simulink model "TransmissionLine"  (R2025a)
settings: Solver=ode15s  StartTime=0.0  StopTime=0.2  RelTol=1e-3
libraries: spsFourierLib x6, dspfdesign x6, spsDistributedParametersLineLib x2, spsThreePhaseVIMeasurementLib x2, spsThreePhaseBreakerLib x2, spsThreePhaseSourceLib x2, simulink_extras x1, spsOnDelayLib x1, spsThreePhaseFaultLib x1, sps_lib x1
settings Model: Creator=monji  LastModifiedBy=monji

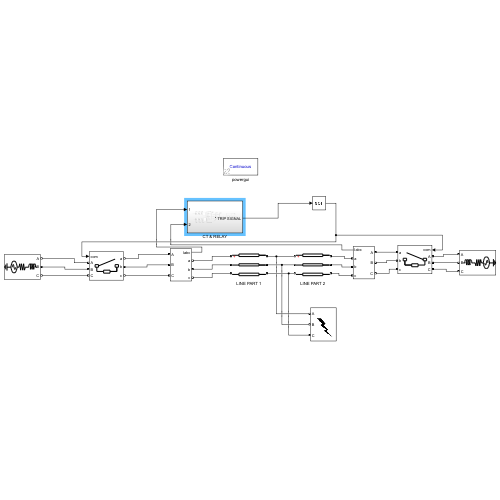
[thumbnail: Simulink's stored preview of the top-level diagram]
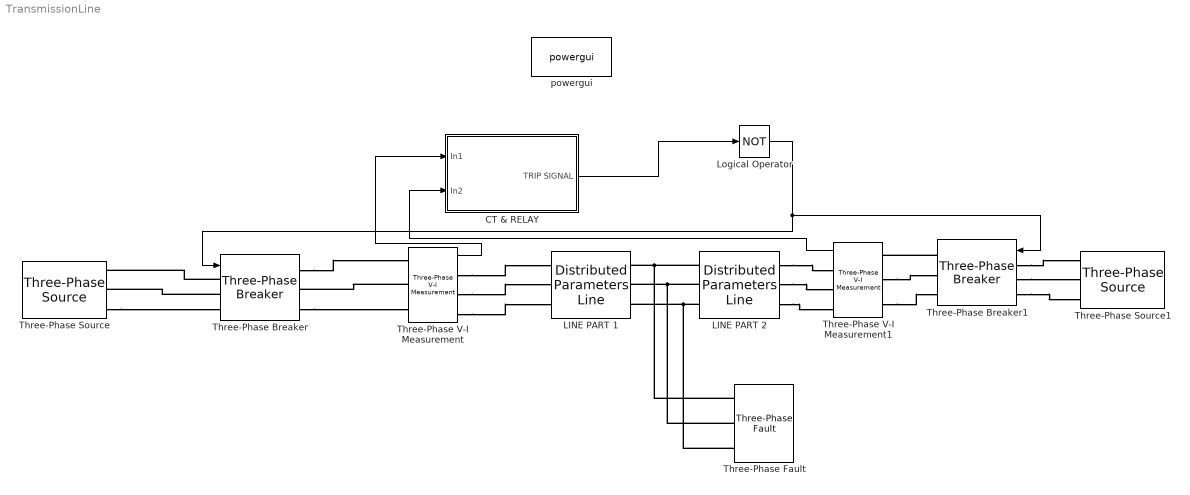
== system TransmissionLine ==
  CT & RELAY : Subsystem
  LINE PART 1 : spsDistributedParametersLineLib/Distributed Parameters Line  Phases=3  Length=10  Frequency=50  Resistance=[0.045531917 0.151489359 ]  Inductance=[0.0006176566224 0.001533982723]  Capacitance=[0.013e-8 0.0085e-8]  x1=[1.46385157011448e-06 84909.030148672 84909.030146414;314.159265358979 314.159265358979 314.159265358979;-0.0832984052830537 0.256881061681218 -1.31391526508876]  x2=[1.4638153564349e-06 84909.0444627924 84909.0444605344;314.159265358979 314.159265358979 314.159265358979;-0.0832705183654309 0.256879998490702 -1.31391632827928]  x3=[3.47740712938383e-10 38.9054582092484 38.90545820819;314.159265358979 314.159265358979 314.159265358979;-0.0653475125454102 0.255989829496242 -1.31480649727325]  x4=[3.43279937985723e-10 38.9903495109087 38.9903495098979;314.159265358979 314.159265358979 314.159265358979;-0.109935333243445 0.256879998680736 -1.31391632808959]  x5=3.61093521757176e-06  V1=[1.464e-06 8.491e+04 8.491e+04;314.2 314.2 314.2;-0.0833 0.2569 -1.314]  V2=[1.464e-06 8.491e+04 8.491e+04;314.2 314.2 314.2;-0.08327 0.2569 -1.314]  I1=[3.477e-10 38.91 38.91;314.2 314.2 314.2;-0.06535 0.256 -1.315]  I2=[3.433e-10 38.99 38.99;314.2 314.2 314.2;-0.1099 0.2569 -1.314]  nHarmo=1  Measurements=None  Decoupling=off  VsMag0=0  VrMag0=0  VsAngle0=0  VrAngle0=0  IsMag0=0  IrMag0=0  IsAngle0=0  IrAngle0=0
      settings: LibrarySourceBlock=sps_lib/Power Grid Elements/Distributed Parameters Line
  LINE PART 2 : spsDistributedParametersLineLib/Distributed Parameters Line  Phases=3  Length=10  Frequency=50  Resistance=[0.045531917 0.151489359 ]  Inductance=[0.0006176566224 0.001533982723]  Capacitance=[0.013e-8 0.0085e-8]  x1=[1.4638153564349e-06 84909.0444627924 84909.0444605344;314.159265358979 314.159265358979 314.159265358979;-0.0832705183654309 0.256879998490702 -1.31391632827928]  x2=[1.46379725002201e-06 84909.0301487049 84909.0301464468;314.159265358979 314.159265358979 314.159265358979;-0.0832565743891926 0.256881061681343 -1.31391526508863]  x3=[3.46588857006348e-10 38.99034951986 38.9903495188265;314.159265358979 314.159265358979 314.159265358979;-0.0822700055886377 0.256879998301002 -1.31391632846952]  x4=[3.4292641339421e-10 38.9054582002993 38.9054581992604;314.159265358979 314.159265358979 314.159265358979;-0.100050154115277 0.255989829876863 -1.31480649689257]  x5=3.61093521757176e-06  V1=[1.464e-06 8.491e+04 8.491e+04;314.2 314.2 314.2;-0.08327 0.2569 -1.314]  V2=[1.464e-06 8.491e+04 8.491e+04;314.2 314.2 314.2;-0.08326 0.2569 -1.314]  I1=[3.466e-10 38.99 38.99;314.2 314.2 314.2;-0.08227 0.2569 -1.314]  I2=[3.429e-10 38.91 38.91;314.2 314.2 314.2;-0.1001 0.256 -1.315]  nHarmo=1  Measurements=None  Decoupling=off  VsMag0=0  VrMag0=0  VsAngle0=0  VrAngle0=0  IsMag0=0  IrMag0=0  IsAngle0=0  IrAngle0=0
      settings: LibrarySourceBlock=sps_lib/Power Grid Elements/Distributed Parameters Line
  Logical Operator : Logic  Operator=NOT  AllPortsSameDT=off  OutDataTypeStr=boolean
  Three-Phase V-I Measurement : spsThreePhaseVIMeasurementLib/Three-Phase V-I Measurement  VoltageMeasurement=no  SetLabelV=off  LabelV=Vabc  Vpu=off  VpuLL=off  CurrentMeasurement=yes  SetLabelI=off  LabelI=Iabc  Ipu=off  Pbase=100e6  Vbase=500e3  OutputType=Complex  PhasorSimulation=off  PSBequivalent=0
  Three-Phase V-I Measurement1 : spsThreePhaseVIMeasurementLib/Three-Phase V-I Measurement  VoltageMeasurement=no  SetLabelV=off  LabelV=Vabc  Vpu=off  VpuLL=off  CurrentMeasurement=yes  SetLabelI=off  LabelI=Iabc  Ipu=off  Pbase=100e6  Vbase=500e3  OutputType=Complex  PhasorSimulation=off  PSBequivalent=0
  Three-Phase Breaker : spsThreePhaseBreakerLib/Three-Phase Breaker  InitialState=open  SwitchA=on  SwitchB=on  SwitchC=on  SwitchTimes="[1/60  5/60]"  External=on  BreakerResistance=0.001  SnubberResistance=1e6  SnubberCapacitance=inf  Measurements=None
  Three-Phase Breaker1 : spsThreePhaseBreakerLib/Three-Phase Breaker  InitialState=open  SwitchA=on  SwitchB=on  SwitchC=on  SwitchTimes="[1/60  5/60]"  External=on  BreakerResistance=0.001  SnubberResistance=1e6  SnubberCapacitance=inf  Measurements=None
  Three-Phase Fault : spsThreePhaseFaultLib/Three-Phase Fault  InitialStates=0  FaultA=off  FaultB=on  FaultC=on  GroundFault=off  SwitchTimes=[0.05 0.1]  External=off  SwitchStatus=NaN  FaultResistance=5  GroundResistance=0.01  SnubberResistance=1e6  SnubberCapacitance=inf  Measurements=None
  Three-Phase Source : spsThreePhaseSourceLib/Three-Phase Source  InternalConnection=Yg  VoltagePhases=off  Voltage=132e3  PhaseAngle=0  Voltage_phases=[25e3 25e3 25e3]/sqrt(3)  PhaseAngles_phases=[0 -120 +120]  Frequency=50  NonIdealSource=on  SpecifyImpedance=on  Resistance=0.8929  Inductance=16.58e-3  ShortCircuitLevel=2e9  BaseVoltage=25e3  XRratio=7  BusType=swing  Pref=10e3  Qref=0  Prefabc=[10e3, 10e3, 10e3]  Qrefabc=[0, 0, 0]  Qmin=-inf  Qmax=inf
  Three-Phase Source1 : spsThreePhaseSourceLib/Three-Phase Source  InternalConnection=Yg  VoltagePhases=off  Voltage=132e3  PhaseAngle=0  Voltage_phases=[25e3 25e3 25e3]/sqrt(3)  PhaseAngles_phases=[0 -120 +120]  Frequency=50  NonIdealSource=on  SpecifyImpedance=on  Resistance=0.8929  Inductance=16.58e-3  ShortCircuitLevel=1e9  BaseVoltage=25e3  XRratio=7  BusType=swing  Pref=10e3  Qref=0  Prefabc=[10e3, 10e3, 10e3]  Qrefabc=[0, 0, 0]  Qmin=-inf  Qmax=inf
  powergui : sps_lib/powergui  Priority=1  SimulationMode=Continuous  SampleTime=50e-6  frequency=60  Iterations=50  frequencyindice=50  Pbase=100e6  ErrMax=1e-4  UnitsV=kV  UnitsW=MW  buscounter=0  FunctionMessages=off  echomessages=off  EnableUseOfTLC=off  CurrentSourceSwitches=off  DisableSnubberDevices=off  DisableRonSwitches=off  DisableVfSwitches=off  DisplayEquations=off  AutomaticDiscreteSolvers=off  SolverType=Tustin/Backward Euler (TBE)  Interpol=off  ExternalGateDelay=off  methode=off  Ts=100  x0status=blocks  SPID=on  SwTol=0  HookPort=off  NonlinearTolerance=1e-4  nMaxIteration=100  ContinueOnMaxIteration=off  RestoreLinks=warning  ResistiveCurrentMeasurement=off  Frange=[0:2:500]  Ylog=off  Xlog=on  ShowGrid=off  save=off  variable=ZData  structure=0  ZoomFFT=off  StartTime=0.0  cycles=1  DisplayStyle=1  fundamental=60  FreqAxis=off  MaxFrequency=1000  frequencyindicesteady=1  RmsSteady=1  display=off
  wires:
  Three-Phase V-I Measurement/1 -> CT & RELAY/1(In1)
  Three-Phase V-I Measurement1/1 -> CT & RELAY/2(In2)
  CT & RELAY/1(TRIP SIGNAL) -> Logical Operator/1
  Logical Operator/1 -> Three-Phase Breaker1/1, Three-Phase Breaker/1
  connections:
  Three-Phase V-I Measurement/RConn1 -- LINE PART 1/LConn1
  Three-Phase V-I Measurement/RConn2 -- LINE PART 1/LConn2
  Three-Phase V-I Measurement/RConn3 -- LINE PART 1/LConn3
  LINE PART 2/LConn1 -- Three-Phase Fault/LConn1 -- LINE PART 1/RConn1
  LINE PART 2/LConn2 -- Three-Phase Fault/LConn2 -- LINE PART 1/RConn2
  LINE PART 2/LConn3 -- Three-Phase Fault/LConn3 -- LINE PART 1/RConn3
  LINE PART 2/RConn1 -- Three-Phase V-I Measurement1/RConn1
  LINE PART 2/RConn2 -- Three-Phase V-I Measurement1/RConn2
  LINE PART 2/RConn3 -- Three-Phase V-I Measurement1/RConn3
  Three-Phase Breaker/LConn1 -- Three-Phase Source/RConn1
  Three-Phase Breaker/LConn2 -- Three-Phase Source/RConn2
  Three-Phase Source/RConn3 -- Three-Phase Breaker/LConn3
  Three-Phase Breaker/RConn1 -- Three-Phase V-I Measurement/LConn1
  Three-Phase V-I Measurement/LConn2 -- Three-Phase Breaker/RConn2
  Three-Phase Breaker/RConn3 -- Three-Phase V-I Measurement/LConn3
  Three-Phase Breaker1/RConn1 -- Three-Phase V-I Measurement1/LConn1
  Three-Phase V-I Measurement1/LConn2 -- Three-Phase Breaker1/RConn2
  Three-Phase V-I Measurement1/LConn3 -- Three-Phase Breaker1/RConn3
  Three-Phase Breaker1/LConn1 -- Three-Phase Source1/RConn1
  Three-Phase Breaker1/LConn2 -- Three-Phase Source1/RConn2
  Three-Phase Breaker1/LConn3 -- Three-Phase Source1/RConn3

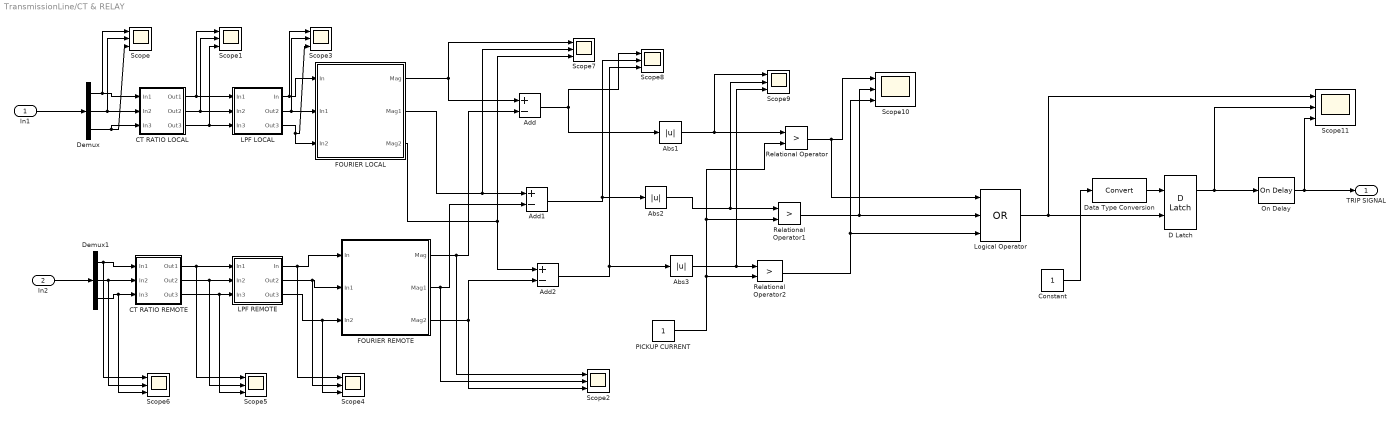
== system TransmissionLine/CT & RELAY ==
  In1 : Inport
  In2 : Inport  Port=2
  Abs1 : Abs  SaturateOnIntegerOverflow=off
  Abs2 : Abs  SaturateOnIntegerOverflow=off
  Abs3 : Abs  SaturateOnIntegerOverflow=off
  Add : Sum  Inputs=+-
  Add1 : Sum  Inputs=+-
  Add2 : Sum  Inputs=+-
  CT RATIO LOCAL : Subsystem
  CT RATIO REMOTE : Subsystem
  Constant : Constant
  D Latch : simulink_extras/Flip Flops/D Latch
  Data Type Conversion : DataTypeConversion  SaturateOnIntegerOverflow=off  RndMeth=Floor
  Demux : Demux  Outputs=3
  Demux1 : Demux  Outputs=3
  FOURIER LOCAL : Subsystem
  FOURIER REMOTE : Subsystem
  LPF LOCAL : Subsystem
  LPF REMOTE : Subsystem
  Logical Operator : Logic  Operator=OR  Inputs=3  AllPortsSameDT=off  OutDataTypeStr=boolean
  On Delay : spsOnDelayLib/On Delay  DelayType=On delay  delay=0.02  ic=0  Ts=0
  PICKUP CURRENT : Constant
  Relational Operator : RelationalOperator  Operator=>  OutDataTypeStr=boolean  RndMeth=Simplest  InputSameDT=off
  Relational Operator1 : RelationalOperator  Operator=>  OutDataTypeStr=boolean  RndMeth=Simplest  InputSameDT=off
  Relational Operator2 : RelationalOperator  Operator=>  OutDataTypeStr=boolean  RndMeth=Simplest  InputSameDT=off
  Scope{,1..11} (12 alike) : Scope  NumInputPorts=3
      Scope settings: ActiveDisplayYMinimum=-18.469678289535427  ActiveDisplayYMaximum=17.061457342627669
      Scope1 settings: ActiveDisplayYMinimum=-1  ActiveDisplayYMaximum=1
      Scope10 settings: ActiveDisplayYMinimum=-0.12499999999999997  ActiveDisplayYMaximum=1.125  DataLoggingVariableName=ScopeData10
      Scope11 settings: ActiveDisplayYMinimum=-0.18459302325581406  ActiveDisplayYMaximum=1.1935319767441861  DataLoggingVariableName=ScopeData11
      Scope2 settings: DataLoggingVariableName=ScopeData2
      Scope3 settings: ActiveDisplayYMinimum=-1  ActiveDisplayYMaximum=1  DataLoggingVariableName=ScopeData3
      Scope4 settings: DataLoggingVariableName=ScopeData4
      Scope5 settings: DataLoggingVariableName=ScopeData5
      Scope6 settings: DataLoggingVariableName=ScopeData6
      Scope7 settings: ActiveDisplayYMinimum=-13.312949145171213  ActiveDisplayYMaximum=119.81654230654095  DataLoggingVariableName=ScopeData7
      Scope8 settings: ActiveDisplayYMinimum=-1  ActiveDisplayYMaximum=1  DataLoggingVariableName=ScopeData8
      Scope9 settings: ActiveDisplayYMinimum=-1.5918447802105358  ActiveDisplayYMaximum=14.326603021894826  DataLoggingVariableName=ScopeData9
  TRIP SIGNAL : Outport
  wires:
  In1/1 -> Demux/1
  In2/1 -> Demux1/1
  Demux/1 -> Scope/1, CT RATIO LOCAL/1(In1)
  Demux/2 -> CT RATIO LOCAL/2(In2), Scope/2
  Demux/3 -> CT RATIO LOCAL/3(In3), Scope/3
  Demux1/1 -> CT RATIO REMOTE/1(In1), Scope6/1
  Demux1/2 -> Scope6/2, CT RATIO REMOTE/2(In2)
  Demux1/3 -> Scope6/3, CT RATIO REMOTE/3(In3)
  CT RATIO LOCAL/1(Out1) -> Scope1/1, LPF LOCAL/1(In1)
  CT RATIO LOCAL/2(Out2) -> Scope1/2, LPF LOCAL/2(In2)
  CT RATIO LOCAL/3(Out3) -> Scope1/3, LPF LOCAL/3(In3)
  CT RATIO REMOTE/1(Out1) -> LPF REMOTE/1(In1), Scope5/1
  CT RATIO REMOTE/2(Out2) -> Scope5/2, LPF REMOTE/2(In2)
  CT RATIO REMOTE/3(Out3) -> Scope5/3, LPF REMOTE/3(In3)
  LPF LOCAL/1(In) -> Scope3/1, FOURIER LOCAL/1(In)
  LPF LOCAL/2(Out2) -> Scope3/2, FOURIER LOCAL/2(In1)
  LPF LOCAL/3(Out3) -> Scope3/3, FOURIER LOCAL/3(In2)
  LPF REMOTE/1(In) -> Scope4/1, FOURIER REMOTE/1(In)
  LPF REMOTE/2(Out2) -> Scope4/2, FOURIER REMOTE/2(In1)
  LPF REMOTE/3(Out3) -> Scope4/3, FOURIER REMOTE/3(In2)
  FOURIER LOCAL/1(Mag) -> Scope7/1, Add/1
  FOURIER REMOTE/1(Mag) -> Scope2/1, Add/2
  FOURIER LOCAL/2(Mag1) -> Scope7/2, Add1/1
  FOURIER REMOTE/2(Mag1) -> Scope2/2, Add1/2
  FOURIER LOCAL/3(Mag2) -> Add2/1, Scope7/3
  FOURIER REMOTE/3(Mag2) -> Add2/2, Scope2/3
  Add/1 -> Scope8/1, Abs1/1
  Add1/1 -> Scope8/2, Abs2/1
  Add2/1 -> Scope8/3, Abs3/1
  Abs1/1 -> Scope9/1, Relational Operator/1
  Abs2/1 -> Scope9/2, Relational Operator1/1
  Abs3/1 -> Scope9/3, Relational Operator2/1
  PICKUP CURRENT/1 -> Relational Operator/2, Relational Operator1/2, Relational Operator2/2
  Relational Operator/1 -> Logical Operator/1, Scope10/1
  Relational Operator1/1 -> Logical Operator/2, Scope10/2
  Relational Operator2/1 -> Logical Operator/3, Scope10/3
  Logical Operator/1 -> Scope11/1, D Latch/2
  Data Type Conversion/1 -> D Latch/1
  Constant/1 -> Data Type Conversion/1
  D Latch/1 -> On Delay/1, Scope11/2
  On Delay/1 -> Scope11/3, TRIP SIGNAL/1

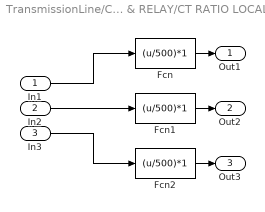
== system TransmissionLine/CT & RELAY/CT RATIO LOCAL ==
  In1 : Inport
  In2 : Inport  Port=2
  In3 : Inport  Port=3
  Fcn : Fcn  Expr=(u/500)*1
  Fcn1 : Fcn  Expr=(u/500)*1
  Fcn2 : Fcn  Expr=(u/500)*1
  Out1 : Outport
  Out2 : Outport  Port=2
  Out3 : Outport  Port=3
  wires:
  In3/1 -> Fcn2/1
  Fcn1/1 -> Out2/1
  In1/1 -> Fcn/1
  Fcn/1 -> Out1/1
  In2/1 -> Fcn1/1
  Fcn2/1 -> Out3/1

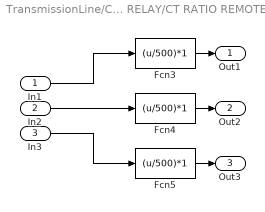
== system TransmissionLine/CT & RELAY/CT RATIO REMOTE ==
  In1 : Inport
  In2 : Inport  Port=2
  In3 : Inport  Port=3
  Fcn3 : Fcn  Expr=(u/500)*1
  Fcn4 : Fcn  Expr=(u/500)*1
  Fcn5 : Fcn  Expr=(u/500)*1
  Out1 : Outport
  Out2 : Outport  Port=2
  Out3 : Outport  Port=3
  wires:
  Fcn5/1 -> Out3/1
  In3/1 -> Fcn5/1
  Fcn3/1 -> Out1/1
  In1/1 -> Fcn3/1
  In2/1 -> Fcn4/1
  Fcn4/1 -> Out2/1

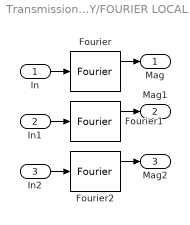
== system TransmissionLine/CT & RELAY/FOURIER LOCAL ==
  In : Inport
  In1 : Inport  Port=2
  In2 : Inport  Port=3
  Fourier : spsFourierLib/Fourier  Freq=50  n=1  InInit=[0, 0]  Ts=0
  Fourier1 : spsFourierLib/Fourier  Freq=50  n=1  InInit=[0, 0]  Ts=0
  Fourier2 : spsFourierLib/Fourier  Freq=50  n=1  InInit=[0, 0]  Ts=0
  Mag : Outport
  Mag1 : Outport  Port=2
  Mag2 : Outport  Port=3
  wires:
  In1/1 -> Fourier1/1
  In/1 -> Fourier/1
  Fourier2/1 -> Mag2/1
  In2/1 -> Fourier2/1
  Fourier1/1 -> Mag1/1
  Fourier/1 -> Mag/1

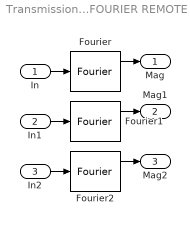
== system TransmissionLine/CT & RELAY/FOURIER REMOTE ==
  In : Inport
  In1 : Inport  Port=2
  In2 : Inport  Port=3
  Fourier : spsFourierLib/Fourier  Freq=50  n=1  InInit=[0, 0]  Ts=0
  Fourier1 : spsFourierLib/Fourier  Freq=50  n=1  InInit=[0, 0]  Ts=0
  Fourier2 : spsFourierLib/Fourier  Freq=50  n=1  InInit=[0, 0]  Ts=0
  Mag : Outport
  Mag1 : Outport  Port=2
  Mag2 : Outport  Port=3
  wires:
  In1/1 -> Fourier1/1
  In/1 -> Fourier/1
  Fourier2/1 -> Mag2/1
  In2/1 -> Fourier2/1
  Fourier1/1 -> Mag1/1
  Fourier/1 -> Mag/1

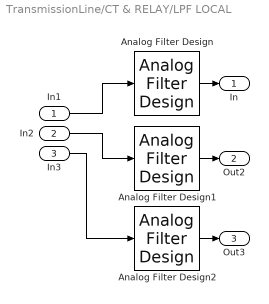
== system TransmissionLine/CT & RELAY/LPF LOCAL ==
  In1 : Inport
  In2 : Inport  Port=2
  In3 : Inport  Port=3
  Analog Filter Design : dspfdesign/Analog Filter Design  method=Butterworth  filttype=Lowpass  N=8  Wlo=500  Whi=80  Rp=2  Rs=40
  Analog Filter Design1 : dspfdesign/Analog Filter Design  method=Butterworth  filttype=Lowpass  N=8  Wlo=500  Whi=80  Rp=2  Rs=40
  Analog Filter Design2 : dspfdesign/Analog Filter Design  method=Butterworth  filttype=Lowpass  N=8  Wlo=500  Whi=80  Rp=2  Rs=40
  In : Outport
  Out2 : Outport  Port=2
  Out3 : Outport  Port=3
  wires:
  Analog Filter Design1/1 -> Out2/1
  In1/1 -> Analog Filter Design/1
  In3/1 -> Analog Filter Design2/1
  Analog Filter Design/1 -> In/1
  Analog Filter Design2/1 -> Out3/1
  In2/1 -> Analog Filter Design1/1

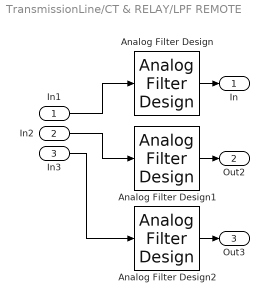
== system TransmissionLine/CT & RELAY/LPF REMOTE ==
  In1 : Inport
  In2 : Inport  Port=2
  In3 : Inport  Port=3
  Analog Filter Design : dspfdesign/Analog Filter Design  method=Butterworth  filttype=Lowpass  N=8  Wlo=500  Whi=80  Rp=2  Rs=40
  Analog Filter Design1 : dspfdesign/Analog Filter Design  method=Butterworth  filttype=Lowpass  N=8  Wlo=500  Whi=80  Rp=2  Rs=40
  Analog Filter Design2 : dspfdesign/Analog Filter Design  method=Butterworth  filttype=Lowpass  N=8  Wlo=500  Whi=80  Rp=2  Rs=40
  In : Outport
  Out2 : Outport  Port=2
  Out3 : Outport  Port=3
  wires:
  Analog Filter Design1/1 -> Out2/1
  In1/1 -> Analog Filter Design/1
  In3/1 -> Analog Filter Design2/1
  Analog Filter Design/1 -> In/1
  Analog Filter Design2/1 -> Out3/1
  In2/1 -> Analog Filter Design1/1
